simulink model "dedisp_sync"  (R2013b)
settings: Solver=FixedStepDiscrete  SolverMode=SingleTasking  StartTime=0.0  StopTime=10.0  RelTol=1e-3
undefined symbols (not defined in the file): pfb_coeff_gen_calc
libraries: xbsIndex_r4 x14646, casper_library_misc x70, casper_library_delays x55, dspsigops x16, xps_library x2, casper_library_pfbs x2
(part 53 of 146)

== system dedisp_sync/Parallel_Dedispersor_v5/Dedispersor_v2_4/detector_block_v212 ==
  Data : Inport
  Valid : Inport  Port=2
  Const1 : xbsIndex_r4/Constant  const=12  gui_display_data_type=Fixed-point  arith_type=Signed (2's comp)  n_bits=16  bin_pt=0  preci_type=Single  exp_width=8  frac_width=24  explicit_period=off  period=1  equ=P=C  opselect=C  inp2=PCIN>>17  opr=+  inp1=P  carry=CIN  dbl_ovrd=off  block_type=constant
  Counter1 : xbsIndex_r4/Counter  cnt_type=Free Running  cnt_to=Inf  operation=Up  start_count=0  cnt_by_val=1  arith_type=Unsigned  n_bits=4  bin_pt=0  load_pin=off  rst=off  en=on  explicit_period=on  period=1  dbl_ovrd=off  use_behavioral_HDL=off  implementation=Fabric  block_type=counter
  Delay1 : xbsIndex_r4/Delay  rst=off  infoeditControl=Selection of Reset will increase slice count due to use of real FFs and instead of SRLs  en=on  latency=13  dbl_ovrd=off  reg_retiming=on  block_type=delay
  Expression1 : xbsIndex_r4/Expression  expression=a & b  align_bp=on  en=off  latency=0  precision=Full  arith_type=Unsigned  n_bits=16  bin_pt=0  dbl_ovrd=off  block_type=expr
  Relational1 : xbsIndex_r4/Relational  mode=a=b  en=off  latency=0  dbl_ovrd=off  block_type=relational
  Out1 : Outport
  wires:
  Valid/1 -> Counter1/1, Expression1/2
  Counter1/1 -> Relational1/1
  Const1/1 -> Relational1/2
  Relational1/1 -> Expression1/1
  Data/1 -> Delay1/1
  Expression1/1 -> Delay1/2
  Delay1/1 -> Out1/1

== system dedisp_sync/Parallel_Dedispersor_v5/Dedispersor_v2_4/detector_block_v213 ==
  Data : Inport
  Valid : Inport  Port=2
  Const1 : xbsIndex_r4/Constant  const=13  gui_display_data_type=Fixed-point  arith_type=Signed (2's comp)  n_bits=16  bin_pt=0  preci_type=Single  exp_width=8  frac_width=24  explicit_period=off  period=1  equ=P=C  opselect=C  inp2=PCIN>>17  opr=+  inp1=P  carry=CIN  dbl_ovrd=off  block_type=constant
  Counter1 : xbsIndex_r4/Counter  cnt_type=Free Running  cnt_to=Inf  operation=Up  start_count=0  cnt_by_val=1  arith_type=Unsigned  n_bits=4  bin_pt=0  load_pin=off  rst=off  en=on  explicit_period=on  period=1  dbl_ovrd=off  use_behavioral_HDL=off  implementation=Fabric  block_type=counter
  Delay1 : xbsIndex_r4/Delay  rst=off  infoeditControl=Selection of Reset will increase slice count due to use of real FFs and instead of SRLs  en=on  latency=14  dbl_ovrd=off  reg_retiming=on  block_type=delay
  Expression1 : xbsIndex_r4/Expression  expression=a & b  align_bp=on  en=off  latency=0  precision=Full  arith_type=Unsigned  n_bits=16  bin_pt=0  dbl_ovrd=off  block_type=expr
  Relational1 : xbsIndex_r4/Relational  mode=a=b  en=off  latency=0  dbl_ovrd=off  block_type=relational
  Out1 : Outport
  wires:
  Valid/1 -> Counter1/1, Expression1/2
  Counter1/1 -> Relational1/1
  Const1/1 -> Relational1/2
  Relational1/1 -> Expression1/1
  Data/1 -> Delay1/1
  Expression1/1 -> Delay1/2
  Delay1/1 -> Out1/1

== system dedisp_sync/Parallel_Dedispersor_v5/Dedispersor_v2_4/detector_block_v214 ==
  Data : Inport
  Valid : Inport  Port=2
  Const1 : xbsIndex_r4/Constant  const=14  gui_display_data_type=Fixed-point  arith_type=Signed (2's comp)  n_bits=16  bin_pt=0  preci_type=Single  exp_width=8  frac_width=24  explicit_period=off  period=1  equ=P=C  opselect=C  inp2=PCIN>>17  opr=+  inp1=P  carry=CIN  dbl_ovrd=off  block_type=constant
  Counter1 : xbsIndex_r4/Counter  cnt_type=Free Running  cnt_to=Inf  operation=Up  start_count=0  cnt_by_val=1  arith_type=Unsigned  n_bits=4  bin_pt=0  load_pin=off  rst=off  en=on  explicit_period=on  period=1  dbl_ovrd=off  use_behavioral_HDL=off  implementation=Fabric  block_type=counter
  Delay1 : xbsIndex_r4/Delay  rst=off  infoeditControl=Selection of Reset will increase slice count due to use of real FFs and instead of SRLs  en=on  latency=15  dbl_ovrd=off  reg_retiming=on  block_type=delay
  Expression1 : xbsIndex_r4/Expression  expression=a & b  align_bp=on  en=off  latency=0  precision=Full  arith_type=Unsigned  n_bits=16  bin_pt=0  dbl_ovrd=off  block_type=expr
  Relational1 : xbsIndex_r4/Relational  mode=a=b  en=off  latency=0  dbl_ovrd=off  block_type=relational
  Out1 : Outport
  wires:
  Valid/1 -> Counter1/1, Expression1/2
  Counter1/1 -> Relational1/1
  Const1/1 -> Relational1/2
  Relational1/1 -> Expression1/1
  Data/1 -> Delay1/1
  Expression1/1 -> Delay1/2
  Delay1/1 -> Out1/1

== system dedisp_sync/Parallel_Dedispersor_v5/Dedispersor_v2_4/detector_block_v215 ==
  Data : Inport
  Valid : Inport  Port=2
  Const1 : xbsIndex_r4/Constant  const=15  gui_display_data_type=Fixed-point  arith_type=Signed (2's comp)  n_bits=16  bin_pt=0  preci_type=Single  exp_width=8  frac_width=24  explicit_period=off  period=1  equ=P=C  opselect=C  inp2=PCIN>>17  opr=+  inp1=P  carry=CIN  dbl_ovrd=off  block_type=constant
  Counter1 : xbsIndex_r4/Counter  cnt_type=Free Running  cnt_to=Inf  operation=Up  start_count=0  cnt_by_val=1  arith_type=Unsigned  n_bits=4  bin_pt=0  load_pin=off  rst=off  en=on  explicit_period=on  period=1  dbl_ovrd=off  use_behavioral_HDL=off  implementation=Fabric  block_type=counter
  Delay1 : xbsIndex_r4/Delay  rst=off  infoeditControl=Selection of Reset will increase slice count due to use of real FFs and instead of SRLs  en=on  latency=16  dbl_ovrd=off  reg_retiming=on  block_type=delay
  Expression1 : xbsIndex_r4/Expression  expression=a & b  align_bp=on  en=off  latency=0  precision=Full  arith_type=Unsigned  n_bits=16  bin_pt=0  dbl_ovrd=off  block_type=expr
  Relational1 : xbsIndex_r4/Relational  mode=a=b  en=off  latency=0  dbl_ovrd=off  block_type=relational
  Out1 : Outport
  wires:
  Valid/1 -> Counter1/1, Expression1/2
  Counter1/1 -> Relational1/1
  Const1/1 -> Relational1/2
  Relational1/1 -> Expression1/1
  Data/1 -> Delay1/1
  Expression1/1 -> Delay1/2
  Delay1/1 -> Out1/1

== system dedisp_sync/Parallel_Dedispersor_v5/Dedispersor_v2_4/detector_block_v22 ==
  Data : Inport
  Valid : Inport  Port=2
  Const1 : xbsIndex_r4/Constant  const=2  gui_display_data_type=Fixed-point  arith_type=Signed (2's comp)  n_bits=16  bin_pt=0  preci_type=Single  exp_width=8  frac_width=24  explicit_period=off  period=1  equ=P=C  opselect=C  inp2=PCIN>>17  opr=+  inp1=P  carry=CIN  dbl_ovrd=off  block_type=constant
  Counter1 : xbsIndex_r4/Counter  cnt_type=Free Running  cnt_to=Inf  operation=Up  start_count=0  cnt_by_val=1  arith_type=Unsigned  n_bits=4  bin_pt=0  load_pin=off  rst=off  en=on  explicit_period=on  period=1  dbl_ovrd=off  use_behavioral_HDL=off  implementation=Fabric  block_type=counter
  Delay1 : xbsIndex_r4/Delay  rst=off  infoeditControl=Selection of Reset will increase slice count due to use of real FFs and instead of SRLs  en=on  latency=3  dbl_ovrd=off  reg_retiming=on  block_type=delay
  Expression1 : xbsIndex_r4/Expression  expression=a & b  align_bp=on  en=off  latency=0  precision=Full  arith_type=Unsigned  n_bits=16  bin_pt=0  dbl_ovrd=off  block_type=expr
  Relational1 : xbsIndex_r4/Relational  mode=a=b  en=off  latency=0  dbl_ovrd=off  block_type=relational
  Out1 : Outport
  wires:
  Valid/1 -> Counter1/1, Expression1/2
  Counter1/1 -> Relational1/1
  Const1/1 -> Relational1/2
  Relational1/1 -> Expression1/1
  Data/1 -> Delay1/1
  Expression1/1 -> Delay1/2
  Delay1/1 -> Out1/1

== system dedisp_sync/Parallel_Dedispersor_v5/Dedispersor_v2_4/detector_block_v23 ==
  Data : Inport
  Valid : Inport  Port=2
  Const1 : xbsIndex_r4/Constant  const=3  gui_display_data_type=Fixed-point  arith_type=Signed (2's comp)  n_bits=16  bin_pt=0  preci_type=Single  exp_width=8  frac_width=24  explicit_period=off  period=1  equ=P=C  opselect=C  inp2=PCIN>>17  opr=+  inp1=P  carry=CIN  dbl_ovrd=off  block_type=constant
  Counter1 : xbsIndex_r4/Counter  cnt_type=Free Running  cnt_to=Inf  operation=Up  start_count=0  cnt_by_val=1  arith_type=Unsigned  n_bits=4  bin_pt=0  load_pin=off  rst=off  en=on  explicit_period=on  period=1  dbl_ovrd=off  use_behavioral_HDL=off  implementation=Fabric  block_type=counter
  Delay1 : xbsIndex_r4/Delay  rst=off  infoeditControl=Selection of Reset will increase slice count due to use of real FFs and instead of SRLs  en=on  latency=4  dbl_ovrd=off  reg_retiming=on  block_type=delay
  Expression1 : xbsIndex_r4/Expression  expression=a & b  align_bp=on  en=off  latency=0  precision=Full  arith_type=Unsigned  n_bits=16  bin_pt=0  dbl_ovrd=off  block_type=expr
  Relational1 : xbsIndex_r4/Relational  mode=a=b  en=off  latency=0  dbl_ovrd=off  block_type=relational
  Out1 : Outport
  wires:
  Valid/1 -> Counter1/1, Expression1/2
  Counter1/1 -> Relational1/1
  Const1/1 -> Relational1/2
  Relational1/1 -> Expression1/1
  Data/1 -> Delay1/1
  Expression1/1 -> Delay1/2
  Delay1/1 -> Out1/1

== system dedisp_sync/Parallel_Dedispersor_v5/Dedispersor_v2_4/detector_block_v24 ==
  Data : Inport
  Valid : Inport  Port=2
  Const1 : xbsIndex_r4/Constant  const=4  gui_display_data_type=Fixed-point  arith_type=Signed (2's comp)  n_bits=16  bin_pt=0  preci_type=Single  exp_width=8  frac_width=24  explicit_period=off  period=1  equ=P=C  opselect=C  inp2=PCIN>>17  opr=+  inp1=P  carry=CIN  dbl_ovrd=off  block_type=constant
  Counter1 : xbsIndex_r4/Counter  cnt_type=Free Running  cnt_to=Inf  operation=Up  start_count=0  cnt_by_val=1  arith_type=Unsigned  n_bits=4  bin_pt=0  load_pin=off  rst=off  en=on  explicit_period=on  period=1  dbl_ovrd=off  use_behavioral_HDL=off  implementation=Fabric  block_type=counter
  Delay1 : xbsIndex_r4/Delay  rst=off  infoeditControl=Selection of Reset will increase slice count due to use of real FFs and instead of SRLs  en=on  latency=5  dbl_ovrd=off  reg_retiming=on  block_type=delay
  Expression1 : xbsIndex_r4/Expression  expression=a & b  align_bp=on  en=off  latency=0  precision=Full  arith_type=Unsigned  n_bits=16  bin_pt=0  dbl_ovrd=off  block_type=expr
  Relational1 : xbsIndex_r4/Relational  mode=a=b  en=off  latency=0  dbl_ovrd=off  block_type=relational
  Out1 : Outport
  wires:
  Valid/1 -> Counter1/1, Expression1/2
  Counter1/1 -> Relational1/1
  Const1/1 -> Relational1/2
  Relational1/1 -> Expression1/1
  Data/1 -> Delay1/1
  Expression1/1 -> Delay1/2
  Delay1/1 -> Out1/1

== system dedisp_sync/Parallel_Dedispersor_v5/Dedispersor_v2_4/detector_block_v25 ==
  Data : Inport
  Valid : Inport  Port=2
  Const1 : xbsIndex_r4/Constant  const=5  gui_display_data_type=Fixed-point  arith_type=Signed (2's comp)  n_bits=16  bin_pt=0  preci_type=Single  exp_width=8  frac_width=24  explicit_period=off  period=1  equ=P=C  opselect=C  inp2=PCIN>>17  opr=+  inp1=P  carry=CIN  dbl_ovrd=off  block_type=constant
  Counter1 : xbsIndex_r4/Counter  cnt_type=Free Running  cnt_to=Inf  operation=Up  start_count=0  cnt_by_val=1  arith_type=Unsigned  n_bits=4  bin_pt=0  load_pin=off  rst=off  en=on  explicit_period=on  period=1  dbl_ovrd=off  use_behavioral_HDL=off  implementation=Fabric  block_type=counter
  Delay1 : xbsIndex_r4/Delay  rst=off  infoeditControl=Selection of Reset will increase slice count due to use of real FFs and instead of SRLs  en=on  latency=6  dbl_ovrd=off  reg_retiming=on  block_type=delay
  Expression1 : xbsIndex_r4/Expression  expression=a & b  align_bp=on  en=off  latency=0  precision=Full  arith_type=Unsigned  n_bits=16  bin_pt=0  dbl_ovrd=off  block_type=expr
  Relational1 : xbsIndex_r4/Relational  mode=a=b  en=off  latency=0  dbl_ovrd=off  block_type=relational
  Out1 : Outport
  wires:
  Valid/1 -> Counter1/1, Expression1/2
  Counter1/1 -> Relational1/1
  Const1/1 -> Relational1/2
  Relational1/1 -> Expression1/1
  Data/1 -> Delay1/1
  Expression1/1 -> Delay1/2
  Delay1/1 -> Out1/1

== system dedisp_sync/Parallel_Dedispersor_v5/Dedispersor_v2_4/detector_block_v26 ==
  Data : Inport
  Valid : Inport  Port=2
  Const1 : xbsIndex_r4/Constant  const=6  gui_display_data_type=Fixed-point  arith_type=Signed (2's comp)  n_bits=16  bin_pt=0  preci_type=Single  exp_width=8  frac_width=24  explicit_period=off  period=1  equ=P=C  opselect=C  inp2=PCIN>>17  opr=+  inp1=P  carry=CIN  dbl_ovrd=off  block_type=constant
  Counter1 : xbsIndex_r4/Counter  cnt_type=Free Running  cnt_to=Inf  operation=Up  start_count=0  cnt_by_val=1  arith_type=Unsigned  n_bits=4  bin_pt=0  load_pin=off  rst=off  en=on  explicit_period=on  period=1  dbl_ovrd=off  use_behavioral_HDL=off  implementation=Fabric  block_type=counter
  Delay1 : xbsIndex_r4/Delay  rst=off  infoeditControl=Selection of Reset will increase slice count due to use of real FFs and instead of SRLs  en=on  latency=7  dbl_ovrd=off  reg_retiming=on  block_type=delay
  Expression1 : xbsIndex_r4/Expression  expression=a & b  align_bp=on  en=off  latency=0  precision=Full  arith_type=Unsigned  n_bits=16  bin_pt=0  dbl_ovrd=off  block_type=expr
  Relational1 : xbsIndex_r4/Relational  mode=a=b  en=off  latency=0  dbl_ovrd=off  block_type=relational
  Out1 : Outport
  wires:
  Valid/1 -> Counter1/1, Expression1/2
  Counter1/1 -> Relational1/1
  Const1/1 -> Relational1/2
  Relational1/1 -> Expression1/1
  Data/1 -> Delay1/1
  Expression1/1 -> Delay1/2
  Delay1/1 -> Out1/1

== system dedisp_sync/Parallel_Dedispersor_v5/Dedispersor_v2_4/detector_block_v27 ==
  Data : Inport
  Valid : Inport  Port=2
  Const1 : xbsIndex_r4/Constant  const=7  gui_display_data_type=Fixed-point  arith_type=Signed (2's comp)  n_bits=16  bin_pt=0  preci_type=Single  exp_width=8  frac_width=24  explicit_period=off  period=1  equ=P=C  opselect=C  inp2=PCIN>>17  opr=+  inp1=P  carry=CIN  dbl_ovrd=off  block_type=constant
  Counter1 : xbsIndex_r4/Counter  cnt_type=Free Running  cnt_to=Inf  operation=Up  start_count=0  cnt_by_val=1  arith_type=Unsigned  n_bits=4  bin_pt=0  load_pin=off  rst=off  en=on  explicit_period=on  period=1  dbl_ovrd=off  use_behavioral_HDL=off  implementation=Fabric  block_type=counter
  Delay1 : xbsIndex_r4/Delay  rst=off  infoeditControl=Selection of Reset will increase slice count due to use of real FFs and instead of SRLs  en=on  latency=8  dbl_ovrd=off  reg_retiming=on  block_type=delay
  Expression1 : xbsIndex_r4/Expression  expression=a & b  align_bp=on  en=off  latency=0  precision=Full  arith_type=Unsigned  n_bits=16  bin_pt=0  dbl_ovrd=off  block_type=expr
  Relational1 : xbsIndex_r4/Relational  mode=a=b  en=off  latency=0  dbl_ovrd=off  block_type=relational
  Out1 : Outport
  wires:
  Valid/1 -> Counter1/1, Expression1/2
  Counter1/1 -> Relational1/1
  Const1/1 -> Relational1/2
  Relational1/1 -> Expression1/1
  Data/1 -> Delay1/1
  Expression1/1 -> Delay1/2
  Delay1/1 -> Out1/1

== system dedisp_sync/Parallel_Dedispersor_v5/Dedispersor_v2_4/detector_block_v28 ==
  Data : Inport
  Valid : Inport  Port=2
  Const1 : xbsIndex_r4/Constant  const=8  gui_display_data_type=Fixed-point  arith_type=Signed (2's comp)  n_bits=16  bin_pt=0  preci_type=Single  exp_width=8  frac_width=24  explicit_period=off  period=1  equ=P=C  opselect=C  inp2=PCIN>>17  opr=+  inp1=P  carry=CIN  dbl_ovrd=off  block_type=constant
  Counter1 : xbsIndex_r4/Counter  cnt_type=Free Running  cnt_to=Inf  operation=Up  start_count=0  cnt_by_val=1  arith_type=Unsigned  n_bits=4  bin_pt=0  load_pin=off  rst=off  en=on  explicit_period=on  period=1  dbl_ovrd=off  use_behavioral_HDL=off  implementation=Fabric  block_type=counter
  Delay1 : xbsIndex_r4/Delay  rst=off  infoeditControl=Selection of Reset will increase slice count due to use of real FFs and instead of SRLs  en=on  latency=9  dbl_ovrd=off  reg_retiming=on  block_type=delay
  Expression1 : xbsIndex_r4/Expression  expression=a & b  align_bp=on  en=off  latency=0  precision=Full  arith_type=Unsigned  n_bits=16  bin_pt=0  dbl_ovrd=off  block_type=expr
  Relational1 : xbsIndex_r4/Relational  mode=a=b  en=off  latency=0  dbl_ovrd=off  block_type=relational
  Out1 : Outport
  wires:
  Valid/1 -> Counter1/1, Expression1/2
  Counter1/1 -> Relational1/1
  Const1/1 -> Relational1/2
  Relational1/1 -> Expression1/1
  Data/1 -> Delay1/1
  Expression1/1 -> Delay1/2
  Delay1/1 -> Out1/1

== system dedisp_sync/Parallel_Dedispersor_v5/Dedispersor_v2_4/detector_block_v29 ==
  Data : Inport
  Valid : Inport  Port=2
  Const1 : xbsIndex_r4/Constant  const=9  gui_display_data_type=Fixed-point  arith_type=Signed (2's comp)  n_bits=16  bin_pt=0  preci_type=Single  exp_width=8  frac_width=24  explicit_period=off  period=1  equ=P=C  opselect=C  inp2=PCIN>>17  opr=+  inp1=P  carry=CIN  dbl_ovrd=off  block_type=constant
  Counter1 : xbsIndex_r4/Counter  cnt_type=Free Running  cnt_to=Inf  operation=Up  start_count=0  cnt_by_val=1  arith_type=Unsigned  n_bits=4  bin_pt=0  load_pin=off  rst=off  en=on  explicit_period=on  period=1  dbl_ovrd=off  use_behavioral_HDL=off  implementation=Fabric  block_type=counter
  Delay1 : xbsIndex_r4/Delay  rst=off  infoeditControl=Selection of Reset will increase slice count due to use of real FFs and instead of SRLs  en=on  latency=10  dbl_ovrd=off  reg_retiming=on  block_type=delay
  Expression1 : xbsIndex_r4/Expression  expression=a & b  align_bp=on  en=off  latency=0  precision=Full  arith_type=Unsigned  n_bits=16  bin_pt=0  dbl_ovrd=off  block_type=expr
  Relational1 : xbsIndex_r4/Relational  mode=a=b  en=off  latency=0  dbl_ovrd=off  block_type=relational
  Out1 : Outport
  wires:
  Valid/1 -> Counter1/1, Expression1/2
  Counter1/1 -> Relational1/1
  Const1/1 -> Relational1/2
  Relational1/1 -> Expression1/1
  Data/1 -> Delay1/1
  Expression1/1 -> Delay1/2
  Delay1/1 -> Out1/1

== system dedisp_sync/Parallel_Dedispersor_v6/Dedispersor_v2_1/detector_block_v2 ==
  Data : Inport
  Valid : Inport  Port=2
  Const1 : xbsIndex_r4/Constant  const=0  gui_display_data_type=Fixed-point  arith_type=Signed (2's comp)  n_bits=16  bin_pt=0  preci_type=Single  exp_width=8  frac_width=24  explicit_period=off  period=1  equ=P=C  opselect=C  inp2=PCIN>>17  opr=+  inp1=P  carry=CIN  dbl_ovrd=off  block_type=constant
  Counter1 : xbsIndex_r4/Counter  cnt_type=Free Running  cnt_to=Inf  operation=Up  start_count=0  cnt_by_val=1  arith_type=Unsigned  n_bits=4  bin_pt=0  load_pin=off  rst=off  en=on  explicit_period=on  period=1  dbl_ovrd=off  use_behavioral_HDL=off  implementation=Fabric  block_type=counter
  Delay1 : xbsIndex_r4/Delay  rst=off  infoeditControl=Selection of Reset will increase slice count due to use of real FFs and instead of SRLs  en=on  latency=1  dbl_ovrd=off  reg_retiming=on  block_type=delay
  Expression1 : xbsIndex_r4/Expression  expression=a & b  align_bp=on  en=off  latency=0  precision=Full  arith_type=Unsigned  n_bits=16  bin_pt=0  dbl_ovrd=off  block_type=expr
  Relational1 : xbsIndex_r4/Relational  mode=a=b  en=off  latency=0  dbl_ovrd=off  block_type=relational
  Out1 : Outport
  wires:
  Valid/1 -> Counter1/1, Expression1/2
  Counter1/1 -> Relational1/1
  Const1/1 -> Relational1/2
  Relational1/1 -> Expression1/1
  Data/1 -> Delay1/1
  Expression1/1 -> Delay1/2
  Delay1/1 -> Out1/1

== system dedisp_sync/Parallel_Dedispersor_v6/Dedispersor_v2_1/detector_block_v21 ==
  Data : Inport
  Valid : Inport  Port=2
  Const1 : xbsIndex_r4/Constant  const=1  gui_display_data_type=Fixed-point  arith_type=Signed (2's comp)  n_bits=16  bin_pt=0  preci_type=Single  exp_width=8  frac_width=24  explicit_period=off  period=1  equ=P=C  opselect=C  inp2=PCIN>>17  opr=+  inp1=P  carry=CIN  dbl_ovrd=off  block_type=constant
  Counter1 : xbsIndex_r4/Counter  cnt_type=Free Running  cnt_to=Inf  operation=Up  start_count=0  cnt_by_val=1  arith_type=Unsigned  n_bits=4  bin_pt=0  load_pin=off  rst=off  en=on  explicit_period=on  period=1  dbl_ovrd=off  use_behavioral_HDL=off  implementation=Fabric  block_type=counter
  Delay1 : xbsIndex_r4/Delay  rst=off  infoeditControl=Selection of Reset will increase slice count due to use of real FFs and instead of SRLs  en=on  latency=2  dbl_ovrd=off  reg_retiming=on  block_type=delay
  Expression1 : xbsIndex_r4/Expression  expression=a & b  align_bp=on  en=off  latency=0  precision=Full  arith_type=Unsigned  n_bits=16  bin_pt=0  dbl_ovrd=off  block_type=expr
  Relational1 : xbsIndex_r4/Relational  mode=a=b  en=off  latency=0  dbl_ovrd=off  block_type=relational
  Out1 : Outport
  wires:
  Valid/1 -> Counter1/1, Expression1/2
  Counter1/1 -> Relational1/1
  Const1/1 -> Relational1/2
  Relational1/1 -> Expression1/1
  Data/1 -> Delay1/1
  Expression1/1 -> Delay1/2
  Delay1/1 -> Out1/1

== system dedisp_sync/Parallel_Dedispersor_v6/Dedispersor_v2_1/detector_block_v210 ==
  Data : Inport
  Valid : Inport  Port=2
  Const1 : xbsIndex_r4/Constant  const=10  gui_display_data_type=Fixed-point  arith_type=Signed (2's comp)  n_bits=16  bin_pt=0  preci_type=Single  exp_width=8  frac_width=24  explicit_period=off  period=1  equ=P=C  opselect=C  inp2=PCIN>>17  opr=+  inp1=P  carry=CIN  dbl_ovrd=off  block_type=constant
  Counter1 : xbsIndex_r4/Counter  cnt_type=Free Running  cnt_to=Inf  operation=Up  start_count=0  cnt_by_val=1  arith_type=Unsigned  n_bits=4  bin_pt=0  load_pin=off  rst=off  en=on  explicit_period=on  period=1  dbl_ovrd=off  use_behavioral_HDL=off  implementation=Fabric  block_type=counter
  Delay1 : xbsIndex_r4/Delay  rst=off  infoeditControl=Selection of Reset will increase slice count due to use of real FFs and instead of SRLs  en=on  latency=11  dbl_ovrd=off  reg_retiming=on  block_type=delay
  Expression1 : xbsIndex_r4/Expression  expression=a & b  align_bp=on  en=off  latency=0  precision=Full  arith_type=Unsigned  n_bits=16  bin_pt=0  dbl_ovrd=off  block_type=expr
  Relational1 : xbsIndex_r4/Relational  mode=a=b  en=off  latency=0  dbl_ovrd=off  block_type=relational
  Out1 : Outport
  wires:
  Valid/1 -> Counter1/1, Expression1/2
  Counter1/1 -> Relational1/1
  Const1/1 -> Relational1/2
  Relational1/1 -> Expression1/1
  Data/1 -> Delay1/1
  Expression1/1 -> Delay1/2
  Delay1/1 -> Out1/1

== system dedisp_sync/Parallel_Dedispersor_v6/Dedispersor_v2_1/detector_block_v211 ==
  Data : Inport
  Valid : Inport  Port=2
  Const1 : xbsIndex_r4/Constant  const=11  gui_display_data_type=Fixed-point  arith_type=Signed (2's comp)  n_bits=16  bin_pt=0  preci_type=Single  exp_width=8  frac_width=24  explicit_period=off  period=1  equ=P=C  opselect=C  inp2=PCIN>>17  opr=+  inp1=P  carry=CIN  dbl_ovrd=off  block_type=constant
  Counter1 : xbsIndex_r4/Counter  cnt_type=Free Running  cnt_to=Inf  operation=Up  start_count=0  cnt_by_val=1  arith_type=Unsigned  n_bits=4  bin_pt=0  load_pin=off  rst=off  en=on  explicit_period=on  period=1  dbl_ovrd=off  use_behavioral_HDL=off  implementation=Fabric  block_type=counter
  Delay1 : xbsIndex_r4/Delay  rst=off  infoeditControl=Selection of Reset will increase slice count due to use of real FFs and instead of SRLs  en=on  latency=12  dbl_ovrd=off  reg_retiming=on  block_type=delay
  Expression1 : xbsIndex_r4/Expression  expression=a & b  align_bp=on  en=off  latency=0  precision=Full  arith_type=Unsigned  n_bits=16  bin_pt=0  dbl_ovrd=off  block_type=expr
  Relational1 : xbsIndex_r4/Relational  mode=a=b  en=off  latency=0  dbl_ovrd=off  block_type=relational
  Out1 : Outport
  wires:
  Valid/1 -> Counter1/1, Expression1/2
  Counter1/1 -> Relational1/1
  Const1/1 -> Relational1/2
  Relational1/1 -> Expression1/1
  Data/1 -> Delay1/1
  Expression1/1 -> Delay1/2
  Delay1/1 -> Out1/1

== system dedisp_sync/Parallel_Dedispersor_v6/Dedispersor_v2_1/detector_block_v212 ==
  Data : Inport
  Valid : Inport  Port=2
  Const1 : xbsIndex_r4/Constant  const=12  gui_display_data_type=Fixed-point  arith_type=Signed (2's comp)  n_bits=16  bin_pt=0  preci_type=Single  exp_width=8  frac_width=24  explicit_period=off  period=1  equ=P=C  opselect=C  inp2=PCIN>>17  opr=+  inp1=P  carry=CIN  dbl_ovrd=off  block_type=constant
  Counter1 : xbsIndex_r4/Counter  cnt_type=Free Running  cnt_to=Inf  operation=Up  start_count=0  cnt_by_val=1  arith_type=Unsigned  n_bits=4  bin_pt=0  load_pin=off  rst=off  en=on  explicit_period=on  period=1  dbl_ovrd=off  use_behavioral_HDL=off  implementation=Fabric  block_type=counter
  Delay1 : xbsIndex_r4/Delay  rst=off  infoeditControl=Selection of Reset will increase slice count due to use of real FFs and instead of SRLs  en=on  latency=13  dbl_ovrd=off  reg_retiming=on  block_type=delay
  Expression1 : xbsIndex_r4/Expression  expression=a & b  align_bp=on  en=off  latency=0  precision=Full  arith_type=Unsigned  n_bits=16  bin_pt=0  dbl_ovrd=off  block_type=expr
  Relational1 : xbsIndex_r4/Relational  mode=a=b  en=off  latency=0  dbl_ovrd=off  block_type=relational
  Out1 : Outport
  wires:
  Valid/1 -> Counter1/1, Expression1/2
  Counter1/1 -> Relational1/1
  Const1/1 -> Relational1/2
  Relational1/1 -> Expression1/1
  Data/1 -> Delay1/1
  Expression1/1 -> Delay1/2
  Delay1/1 -> Out1/1

== system dedisp_sync/Parallel_Dedispersor_v6/Dedispersor_v2_1/detector_block_v213 ==
  Data : Inport
  Valid : Inport  Port=2
  Const1 : xbsIndex_r4/Constant  const=13  gui_display_data_type=Fixed-point  arith_type=Signed (2's comp)  n_bits=16  bin_pt=0  preci_type=Single  exp_width=8  frac_width=24  explicit_period=off  period=1  equ=P=C  opselect=C  inp2=PCIN>>17  opr=+  inp1=P  carry=CIN  dbl_ovrd=off  block_type=constant
  Counter1 : xbsIndex_r4/Counter  cnt_type=Free Running  cnt_to=Inf  operation=Up  start_count=0  cnt_by_val=1  arith_type=Unsigned  n_bits=4  bin_pt=0  load_pin=off  rst=off  en=on  explicit_period=on  period=1  dbl_ovrd=off  use_behavioral_HDL=off  implementation=Fabric  block_type=counter
  Delay1 : xbsIndex_r4/Delay  rst=off  infoeditControl=Selection of Reset will increase slice count due to use of real FFs and instead of SRLs  en=on  latency=14  dbl_ovrd=off  reg_retiming=on  block_type=delay
  Expression1 : xbsIndex_r4/Expression  expression=a & b  align_bp=on  en=off  latency=0  precision=Full  arith_type=Unsigned  n_bits=16  bin_pt=0  dbl_ovrd=off  block_type=expr
  Relational1 : xbsIndex_r4/Relational  mode=a=b  en=off  latency=0  dbl_ovrd=off  block_type=relational
  Out1 : Outport
  wires:
  Valid/1 -> Counter1/1, Expression1/2
  Counter1/1 -> Relational1/1
  Const1/1 -> Relational1/2
  Relational1/1 -> Expression1/1
  Data/1 -> Delay1/1
  Expression1/1 -> Delay1/2
  Delay1/1 -> Out1/1

== system dedisp_sync/Parallel_Dedispersor_v6/Dedispersor_v2_1/detector_block_v214 ==
  Data : Inport
  Valid : Inport  Port=2
  Const1 : xbsIndex_r4/Constant  const=14  gui_display_data_type=Fixed-point  arith_type=Signed (2's comp)  n_bits=16  bin_pt=0  preci_type=Single  exp_width=8  frac_width=24  explicit_period=off  period=1  equ=P=C  opselect=C  inp2=PCIN>>17  opr=+  inp1=P  carry=CIN  dbl_ovrd=off  block_type=constant
  Counter1 : xbsIndex_r4/Counter  cnt_type=Free Running  cnt_to=Inf  operation=Up  start_count=0  cnt_by_val=1  arith_type=Unsigned  n_bits=4  bin_pt=0  load_pin=off  rst=off  en=on  explicit_period=on  period=1  dbl_ovrd=off  use_behavioral_HDL=off  implementation=Fabric  block_type=counter
  Delay1 : xbsIndex_r4/Delay  rst=off  infoeditControl=Selection of Reset will increase slice count due to use of real FFs and instead of SRLs  en=on  latency=15  dbl_ovrd=off  reg_retiming=on  block_type=delay
  Expression1 : xbsIndex_r4/Expression  expression=a & b  align_bp=on  en=off  latency=0  precision=Full  arith_type=Unsigned  n_bits=16  bin_pt=0  dbl_ovrd=off  block_type=expr
  Relational1 : xbsIndex_r4/Relational  mode=a=b  en=off  latency=0  dbl_ovrd=off  block_type=relational
  Out1 : Outport
  wires:
  Valid/1 -> Counter1/1, Expression1/2
  Counter1/1 -> Relational1/1
  Const1/1 -> Relational1/2
  Relational1/1 -> Expression1/1
  Data/1 -> Delay1/1
  Expression1/1 -> Delay1/2
  Delay1/1 -> Out1/1

== system dedisp_sync/Parallel_Dedispersor_v6/Dedispersor_v2_1/detector_block_v215 ==
  Data : Inport
  Valid : Inport  Port=2
  Const1 : xbsIndex_r4/Constant  const=15  gui_display_data_type=Fixed-point  arith_type=Signed (2's comp)  n_bits=16  bin_pt=0  preci_type=Single  exp_width=8  frac_width=24  explicit_period=off  period=1  equ=P=C  opselect=C  inp2=PCIN>>17  opr=+  inp1=P  carry=CIN  dbl_ovrd=off  block_type=constant
  Counter1 : xbsIndex_r4/Counter  cnt_type=Free Running  cnt_to=Inf  operation=Up  start_count=0  cnt_by_val=1  arith_type=Unsigned  n_bits=4  bin_pt=0  load_pin=off  rst=off  en=on  explicit_period=on  period=1  dbl_ovrd=off  use_behavioral_HDL=off  implementation=Fabric  block_type=counter
  Delay1 : xbsIndex_r4/Delay  rst=off  infoeditControl=Selection of Reset will increase slice count due to use of real FFs and instead of SRLs  en=on  latency=16  dbl_ovrd=off  reg_retiming=on  block_type=delay
  Expression1 : xbsIndex_r4/Expression  expression=a & b  align_bp=on  en=off  latency=0  precision=Full  arith_type=Unsigned  n_bits=16  bin_pt=0  dbl_ovrd=off  block_type=expr
  Relational1 : xbsIndex_r4/Relational  mode=a=b  en=off  latency=0  dbl_ovrd=off  block_type=relational
  Out1 : Outport
  wires:
  Valid/1 -> Counter1/1, Expression1/2
  Counter1/1 -> Relational1/1
  Const1/1 -> Relational1/2
  Relational1/1 -> Expression1/1
  Data/1 -> Delay1/1
  Expression1/1 -> Delay1/2
  Delay1/1 -> Out1/1

== system dedisp_sync/Parallel_Dedispersor_v6/Dedispersor_v2_1/detector_block_v22 ==
  Data : Inport
  Valid : Inport  Port=2
  Const1 : xbsIndex_r4/Constant  const=2  gui_display_data_type=Fixed-point  arith_type=Signed (2's comp)  n_bits=16  bin_pt=0  preci_type=Single  exp_width=8  frac_width=24  explicit_period=off  period=1  equ=P=C  opselect=C  inp2=PCIN>>17  opr=+  inp1=P  carry=CIN  dbl_ovrd=off  block_type=constant
  Counter1 : xbsIndex_r4/Counter  cnt_type=Free Running  cnt_to=Inf  operation=Up  start_count=0  cnt_by_val=1  arith_type=Unsigned  n_bits=4  bin_pt=0  load_pin=off  rst=off  en=on  explicit_period=on  period=1  dbl_ovrd=off  use_behavioral_HDL=off  implementation=Fabric  block_type=counter
  Delay1 : xbsIndex_r4/Delay  rst=off  infoeditControl=Selection of Reset will increase slice count due to use of real FFs and instead of SRLs  en=on  latency=3  dbl_ovrd=off  reg_retiming=on  block_type=delay
  Expression1 : xbsIndex_r4/Expression  expression=a & b  align_bp=on  en=off  latency=0  precision=Full  arith_type=Unsigned  n_bits=16  bin_pt=0  dbl_ovrd=off  block_type=expr
  Relational1 : xbsIndex_r4/Relational  mode=a=b  en=off  latency=0  dbl_ovrd=off  block_type=relational
  Out1 : Outport
  wires:
  Valid/1 -> Counter1/1, Expression1/2
  Counter1/1 -> Relational1/1
  Const1/1 -> Relational1/2
  Relational1/1 -> Expression1/1
  Data/1 -> Delay1/1
  Expression1/1 -> Delay1/2
  Delay1/1 -> Out1/1

== system dedisp_sync/Parallel_Dedispersor_v6/Dedispersor_v2_1/detector_block_v23 ==
  Data : Inport
  Valid : Inport  Port=2
  Const1 : xbsIndex_r4/Constant  const=3  gui_display_data_type=Fixed-point  arith_type=Signed (2's comp)  n_bits=16  bin_pt=0  preci_type=Single  exp_width=8  frac_width=24  explicit_period=off  period=1  equ=P=C  opselect=C  inp2=PCIN>>17  opr=+  inp1=P  carry=CIN  dbl_ovrd=off  block_type=constant
  Counter1 : xbsIndex_r4/Counter  cnt_type=Free Running  cnt_to=Inf  operation=Up  start_count=0  cnt_by_val=1  arith_type=Unsigned  n_bits=4  bin_pt=0  load_pin=off  rst=off  en=on  explicit_period=on  period=1  dbl_ovrd=off  use_behavioral_HDL=off  implementation=Fabric  block_type=counter
  Delay1 : xbsIndex_r4/Delay  rst=off  infoeditControl=Selection of Reset will increase slice count due to use of real FFs and instead of SRLs  en=on  latency=4  dbl_ovrd=off  reg_retiming=on  block_type=delay
  Expression1 : xbsIndex_r4/Expression  expression=a & b  align_bp=on  en=off  latency=0  precision=Full  arith_type=Unsigned  n_bits=16  bin_pt=0  dbl_ovrd=off  block_type=expr
  Relational1 : xbsIndex_r4/Relational  mode=a=b  en=off  latency=0  dbl_ovrd=off  block_type=relational
  Out1 : Outport
  wires:
  Valid/1 -> Counter1/1, Expression1/2
  Counter1/1 -> Relational1/1
  Const1/1 -> Relational1/2
  Relational1/1 -> Expression1/1
  Data/1 -> Delay1/1
  Expression1/1 -> Delay1/2
  Delay1/1 -> Out1/1

== system dedisp_sync/Parallel_Dedispersor_v6/Dedispersor_v2_1/detector_block_v24 ==
  Data : Inport
  Valid : Inport  Port=2
  Const1 : xbsIndex_r4/Constant  const=4  gui_display_data_type=Fixed-point  arith_type=Signed (2's comp)  n_bits=16  bin_pt=0  preci_type=Single  exp_width=8  frac_width=24  explicit_period=off  period=1  equ=P=C  opselect=C  inp2=PCIN>>17  opr=+  inp1=P  carry=CIN  dbl_ovrd=off  block_type=constant
  Counter1 : xbsIndex_r4/Counter  cnt_type=Free Running  cnt_to=Inf  operation=Up  start_count=0  cnt_by_val=1  arith_type=Unsigned  n_bits=4  bin_pt=0  load_pin=off  rst=off  en=on  explicit_period=on  period=1  dbl_ovrd=off  use_behavioral_HDL=off  implementation=Fabric  block_type=counter
  Delay1 : xbsIndex_r4/Delay  rst=off  infoeditControl=Selection of Reset will increase slice count due to use of real FFs and instead of SRLs  en=on  latency=5  dbl_ovrd=off  reg_retiming=on  block_type=delay
  Expression1 : xbsIndex_r4/Expression  expression=a & b  align_bp=on  en=off  latency=0  precision=Full  arith_type=Unsigned  n_bits=16  bin_pt=0  dbl_ovrd=off  block_type=expr
  Relational1 : xbsIndex_r4/Relational  mode=a=b  en=off  latency=0  dbl_ovrd=off  block_type=relational
  Out1 : Outport
  wires:
  Valid/1 -> Counter1/1, Expression1/2
  Counter1/1 -> Relational1/1
  Const1/1 -> Relational1/2
  Relational1/1 -> Expression1/1
  Data/1 -> Delay1/1
  Expression1/1 -> Delay1/2
  Delay1/1 -> Out1/1

== system dedisp_sync/Parallel_Dedispersor_v6/Dedispersor_v2_1/detector_block_v25 ==
  Data : Inport
  Valid : Inport  Port=2
  Const1 : xbsIndex_r4/Constant  const=5  gui_display_data_type=Fixed-point  arith_type=Signed (2's comp)  n_bits=16  bin_pt=0  preci_type=Single  exp_width=8  frac_width=24  explicit_period=off  period=1  equ=P=C  opselect=C  inp2=PCIN>>17  opr=+  inp1=P  carry=CIN  dbl_ovrd=off  block_type=constant
  Counter1 : xbsIndex_r4/Counter  cnt_type=Free Running  cnt_to=Inf  operation=Up  start_count=0  cnt_by_val=1  arith_type=Unsigned  n_bits=4  bin_pt=0  load_pin=off  rst=off  en=on  explicit_period=on  period=1  dbl_ovrd=off  use_behavioral_HDL=off  implementation=Fabric  block_type=counter
  Delay1 : xbsIndex_r4/Delay  rst=off  infoeditControl=Selection of Reset will increase slice count due to use of real FFs and instead of SRLs  en=on  latency=6  dbl_ovrd=off  reg_retiming=on  block_type=delay
  Expression1 : xbsIndex_r4/Expression  expression=a & b  align_bp=on  en=off  latency=0  precision=Full  arith_type=Unsigned  n_bits=16  bin_pt=0  dbl_ovrd=off  block_type=expr
  Relational1 : xbsIndex_r4/Relational  mode=a=b  en=off  latency=0  dbl_ovrd=off  block_type=relational
  Out1 : Outport
  wires:
  Valid/1 -> Counter1/1, Expression1/2
  Counter1/1 -> Relational1/1
  Const1/1 -> Relational1/2
  Relational1/1 -> Expression1/1
  Data/1 -> Delay1/1
  Expression1/1 -> Delay1/2
  Delay1/1 -> Out1/1

== system dedisp_sync/Parallel_Dedispersor_v6/Dedispersor_v2_1/detector_block_v26 ==
  Data : Inport
  Valid : Inport  Port=2
  Const1 : xbsIndex_r4/Constant  const=6  gui_display_data_type=Fixed-point  arith_type=Signed (2's comp)  n_bits=16  bin_pt=0  preci_type=Single  exp_width=8  frac_width=24  explicit_period=off  period=1  equ=P=C  opselect=C  inp2=PCIN>>17  opr=+  inp1=P  carry=CIN  dbl_ovrd=off  block_type=constant
  Counter1 : xbsIndex_r4/Counter  cnt_type=Free Running  cnt_to=Inf  operation=Up  start_count=0  cnt_by_val=1  arith_type=Unsigned  n_bits=4  bin_pt=0  load_pin=off  rst=off  en=on  explicit_period=on  period=1  dbl_ovrd=off  use_behavioral_HDL=off  implementation=Fabric  block_type=counter
  Delay1 : xbsIndex_r4/Delay  rst=off  infoeditControl=Selection of Reset will increase slice count due to use of real FFs and instead of SRLs  en=on  latency=7  dbl_ovrd=off  reg_retiming=on  block_type=delay
  Expression1 : xbsIndex_r4/Expression  expression=a & b  align_bp=on  en=off  latency=0  precision=Full  arith_type=Unsigned  n_bits=16  bin_pt=0  dbl_ovrd=off  block_type=expr
  Relational1 : xbsIndex_r4/Relational  mode=a=b  en=off  latency=0  dbl_ovrd=off  block_type=relational
  Out1 : Outport
  wires:
  Valid/1 -> Counter1/1, Expression1/2
  Counter1/1 -> Relational1/1
  Const1/1 -> Relational1/2
  Relational1/1 -> Expression1/1
  Data/1 -> Delay1/1
  Expression1/1 -> Delay1/2
  Delay1/1 -> Out1/1

== system dedisp_sync/Parallel_Dedispersor_v6/Dedispersor_v2_1/detector_block_v27 ==
  Data : Inport
  Valid : Inport  Port=2
  Const1 : xbsIndex_r4/Constant  const=7  gui_display_data_type=Fixed-point  arith_type=Signed (2's comp)  n_bits=16  bin_pt=0  preci_type=Single  exp_width=8  frac_width=24  explicit_period=off  period=1  equ=P=C  opselect=C  inp2=PCIN>>17  opr=+  inp1=P  carry=CIN  dbl_ovrd=off  block_type=constant
  Counter1 : xbsIndex_r4/Counter  cnt_type=Free Running  cnt_to=Inf  operation=Up  start_count=0  cnt_by_val=1  arith_type=Unsigned  n_bits=4  bin_pt=0  load_pin=off  rst=off  en=on  explicit_period=on  period=1  dbl_ovrd=off  use_behavioral_HDL=off  implementation=Fabric  block_type=counter
  Delay1 : xbsIndex_r4/Delay  rst=off  infoeditControl=Selection of Reset will increase slice count due to use of real FFs and instead of SRLs  en=on  latency=8  dbl_ovrd=off  reg_retiming=on  block_type=delay
  Expression1 : xbsIndex_r4/Expression  expression=a & b  align_bp=on  en=off  latency=0  precision=Full  arith_type=Unsigned  n_bits=16  bin_pt=0  dbl_ovrd=off  block_type=expr
  Relational1 : xbsIndex_r4/Relational  mode=a=b  en=off  latency=0  dbl_ovrd=off  block_type=relational
  Out1 : Outport
  wires:
  Valid/1 -> Counter1/1, Expression1/2
  Counter1/1 -> Relational1/1
  Const1/1 -> Relational1/2
  Relational1/1 -> Expression1/1
  Data/1 -> Delay1/1
  Expression1/1 -> Delay1/2
  Delay1/1 -> Out1/1

== system dedisp_sync/Parallel_Dedispersor_v6/Dedispersor_v2_1/detector_block_v28 ==
  Data : Inport
  Valid : Inport  Port=2
  Const1 : xbsIndex_r4/Constant  const=8  gui_display_data_type=Fixed-point  arith_type=Signed (2's comp)  n_bits=16  bin_pt=0  preci_type=Single  exp_width=8  frac_width=24  explicit_period=off  period=1  equ=P=C  opselect=C  inp2=PCIN>>17  opr=+  inp1=P  carry=CIN  dbl_ovrd=off  block_type=constant
  Counter1 : xbsIndex_r4/Counter  cnt_type=Free Running  cnt_to=Inf  operation=Up  start_count=0  cnt_by_val=1  arith_type=Unsigned  n_bits=4  bin_pt=0  load_pin=off  rst=off  en=on  explicit_period=on  period=1  dbl_ovrd=off  use_behavioral_HDL=off  implementation=Fabric  block_type=counter
  Delay1 : xbsIndex_r4/Delay  rst=off  infoeditControl=Selection of Reset will increase slice count due to use of real FFs and instead of SRLs  en=on  latency=9  dbl_ovrd=off  reg_retiming=on  block_type=delay
  Expression1 : xbsIndex_r4/Expression  expression=a & b  align_bp=on  en=off  latency=0  precision=Full  arith_type=Unsigned  n_bits=16  bin_pt=0  dbl_ovrd=off  block_type=expr
  Relational1 : xbsIndex_r4/Relational  mode=a=b  en=off  latency=0  dbl_ovrd=off  block_type=relational
  Out1 : Outport
  wires:
  Valid/1 -> Counter1/1, Expression1/2
  Counter1/1 -> Relational1/1
  Const1/1 -> Relational1/2
  Relational1/1 -> Expression1/1
  Data/1 -> Delay1/1
  Expression1/1 -> Delay1/2
  Delay1/1 -> Out1/1

== system dedisp_sync/Parallel_Dedispersor_v6/Dedispersor_v2_1/detector_block_v29 ==
  Data : Inport
  Valid : Inport  Port=2
  Const1 : xbsIndex_r4/Constant  const=9  gui_display_data_type=Fixed-point  arith_type=Signed (2's comp)  n_bits=16  bin_pt=0  preci_type=Single  exp_width=8  frac_width=24  explicit_period=off  period=1  equ=P=C  opselect=C  inp2=PCIN>>17  opr=+  inp1=P  carry=CIN  dbl_ovrd=off  block_type=constant
  Counter1 : xbsIndex_r4/Counter  cnt_type=Free Running  cnt_to=Inf  operation=Up  start_count=0  cnt_by_val=1  arith_type=Unsigned  n_bits=4  bin_pt=0  load_pin=off  rst=off  en=on  explicit_period=on  period=1  dbl_ovrd=off  use_behavioral_HDL=off  implementation=Fabric  block_type=counter
  Delay1 : xbsIndex_r4/Delay  rst=off  infoeditControl=Selection of Reset will increase slice count due to use of real FFs and instead of SRLs  en=on  latency=10  dbl_ovrd=off  reg_retiming=on  block_type=delay
  Expression1 : xbsIndex_r4/Expression  expression=a & b  align_bp=on  en=off  latency=0  precision=Full  arith_type=Unsigned  n_bits=16  bin_pt=0  dbl_ovrd=off  block_type=expr
  Relational1 : xbsIndex_r4/Relational  mode=a=b  en=off  latency=0  dbl_ovrd=off  block_type=relational
  Out1 : Outport
  wires:
  Valid/1 -> Counter1/1, Expression1/2
  Counter1/1 -> Relational1/1
  Const1/1 -> Relational1/2
  Relational1/1 -> Expression1/1
  Data/1 -> Delay1/1
  Expression1/1 -> Delay1/2
  Delay1/1 -> Out1/1

== system dedisp_sync/Parallel_Dedispersor_v6/Dedispersor_v2_2/detector_block_v2 ==
  Data : Inport
  Valid : Inport  Port=2
  Const1 : xbsIndex_r4/Constant  const=0  gui_display_data_type=Fixed-point  arith_type=Signed (2's comp)  n_bits=16  bin_pt=0  preci_type=Single  exp_width=8  frac_width=24  explicit_period=off  period=1  equ=P=C  opselect=C  inp2=PCIN>>17  opr=+  inp1=P  carry=CIN  dbl_ovrd=off  block_type=constant
  Counter1 : xbsIndex_r4/Counter  cnt_type=Free Running  cnt_to=Inf  operation=Up  start_count=0  cnt_by_val=1  arith_type=Unsigned  n_bits=4  bin_pt=0  load_pin=off  rst=off  en=on  explicit_period=on  period=1  dbl_ovrd=off  use_behavioral_HDL=off  implementation=Fabric  block_type=counter
  Delay1 : xbsIndex_r4/Delay  rst=off  infoeditControl=Selection of Reset will increase slice count due to use of real FFs and instead of SRLs  en=on  latency=1  dbl_ovrd=off  reg_retiming=on  block_type=delay
  Expression1 : xbsIndex_r4/Expression  expression=a & b  align_bp=on  en=off  latency=0  precision=Full  arith_type=Unsigned  n_bits=16  bin_pt=0  dbl_ovrd=off  block_type=expr
  Relational1 : xbsIndex_r4/Relational  mode=a=b  en=off  latency=0  dbl_ovrd=off  block_type=relational
  Out1 : Outport
  wires:
  Valid/1 -> Counter1/1, Expression1/2
  Counter1/1 -> Relational1/1
  Const1/1 -> Relational1/2
  Relational1/1 -> Expression1/1
  Data/1 -> Delay1/1
  Expression1/1 -> Delay1/2
  Delay1/1 -> Out1/1

== system dedisp_sync/Parallel_Dedispersor_v6/Dedispersor_v2_2/detector_block_v21 ==
  Data : Inport
  Valid : Inport  Port=2
  Const1 : xbsIndex_r4/Constant  const=1  gui_display_data_type=Fixed-point  arith_type=Signed (2's comp)  n_bits=16  bin_pt=0  preci_type=Single  exp_width=8  frac_width=24  explicit_period=off  period=1  equ=P=C  opselect=C  inp2=PCIN>>17  opr=+  inp1=P  carry=CIN  dbl_ovrd=off  block_type=constant
  Counter1 : xbsIndex_r4/Counter  cnt_type=Free Running  cnt_to=Inf  operation=Up  start_count=0  cnt_by_val=1  arith_type=Unsigned  n_bits=4  bin_pt=0  load_pin=off  rst=off  en=on  explicit_period=on  period=1  dbl_ovrd=off  use_behavioral_HDL=off  implementation=Fabric  block_type=counter
  Delay1 : xbsIndex_r4/Delay  rst=off  infoeditControl=Selection of Reset will increase slice count due to use of real FFs and instead of SRLs  en=on  latency=2  dbl_ovrd=off  reg_retiming=on  block_type=delay
  Expression1 : xbsIndex_r4/Expression  expression=a & b  align_bp=on  en=off  latency=0  precision=Full  arith_type=Unsigned  n_bits=16  bin_pt=0  dbl_ovrd=off  block_type=expr
  Relational1 : xbsIndex_r4/Relational  mode=a=b  en=off  latency=0  dbl_ovrd=off  block_type=relational
  Out1 : Outport
  wires:
  Valid/1 -> Counter1/1, Expression1/2
  Counter1/1 -> Relational1/1
  Const1/1 -> Relational1/2
  Relational1/1 -> Expression1/1
  Data/1 -> Delay1/1
  Expression1/1 -> Delay1/2
  Delay1/1 -> Out1/1

== system dedisp_sync/Parallel_Dedispersor_v6/Dedispersor_v2_2/detector_block_v210 ==
  Data : Inport
  Valid : Inport  Port=2
  Const1 : xbsIndex_r4/Constant  const=10  gui_display_data_type=Fixed-point  arith_type=Signed (2's comp)  n_bits=16  bin_pt=0  preci_type=Single  exp_width=8  frac_width=24  explicit_period=off  period=1  equ=P=C  opselect=C  inp2=PCIN>>17  opr=+  inp1=P  carry=CIN  dbl_ovrd=off  block_type=constant
  Counter1 : xbsIndex_r4/Counter  cnt_type=Free Running  cnt_to=Inf  operation=Up  start_count=0  cnt_by_val=1  arith_type=Unsigned  n_bits=4  bin_pt=0  load_pin=off  rst=off  en=on  explicit_period=on  period=1  dbl_ovrd=off  use_behavioral_HDL=off  implementation=Fabric  block_type=counter
  Delay1 : xbsIndex_r4/Delay  rst=off  infoeditControl=Selection of Reset will increase slice count due to use of real FFs and instead of SRLs  en=on  latency=11  dbl_ovrd=off  reg_retiming=on  block_type=delay
  Expression1 : xbsIndex_r4/Expression  expression=a & b  align_bp=on  en=off  latency=0  precision=Full  arith_type=Unsigned  n_bits=16  bin_pt=0  dbl_ovrd=off  block_type=expr
  Relational1 : xbsIndex_r4/Relational  mode=a=b  en=off  latency=0  dbl_ovrd=off  block_type=relational
  Out1 : Outport
  wires:
  Valid/1 -> Counter1/1, Expression1/2
  Counter1/1 -> Relational1/1
  Const1/1 -> Relational1/2
  Relational1/1 -> Expression1/1
  Data/1 -> Delay1/1
  Expression1/1 -> Delay1/2
  Delay1/1 -> Out1/1

== system dedisp_sync/Parallel_Dedispersor_v6/Dedispersor_v2_2/detector_block_v211 ==
  Data : Inport
  Valid : Inport  Port=2
  Const1 : xbsIndex_r4/Constant  const=11  gui_display_data_type=Fixed-point  arith_type=Signed (2's comp)  n_bits=16  bin_pt=0  preci_type=Single  exp_width=8  frac_width=24  explicit_period=off  period=1  equ=P=C  opselect=C  inp2=PCIN>>17  opr=+  inp1=P  carry=CIN  dbl_ovrd=off  block_type=constant
  Counter1 : xbsIndex_r4/Counter  cnt_type=Free Running  cnt_to=Inf  operation=Up  start_count=0  cnt_by_val=1  arith_type=Unsigned  n_bits=4  bin_pt=0  load_pin=off  rst=off  en=on  explicit_period=on  period=1  dbl_ovrd=off  use_behavioral_HDL=off  implementation=Fabric  block_type=counter
  Delay1 : xbsIndex_r4/Delay  rst=off  infoeditControl=Selection of Reset will increase slice count due to use of real FFs and instead of SRLs  en=on  latency=12  dbl_ovrd=off  reg_retiming=on  block_type=delay
  Expression1 : xbsIndex_r4/Expression  expression=a & b  align_bp=on  en=off  latency=0  precision=Full  arith_type=Unsigned  n_bits=16  bin_pt=0  dbl_ovrd=off  block_type=expr
  Relational1 : xbsIndex_r4/Relational  mode=a=b  en=off  latency=0  dbl_ovrd=off  block_type=relational
  Out1 : Outport
  wires:
  Valid/1 -> Counter1/1, Expression1/2
  Counter1/1 -> Relational1/1
  Const1/1 -> Relational1/2
  Relational1/1 -> Expression1/1
  Data/1 -> Delay1/1
  Expression1/1 -> Delay1/2
  Delay1/1 -> Out1/1

== system dedisp_sync/Parallel_Dedispersor_v6/Dedispersor_v2_2/detector_block_v212 ==
  Data : Inport
  Valid : Inport  Port=2
  Const1 : xbsIndex_r4/Constant  const=12  gui_display_data_type=Fixed-point  arith_type=Signed (2's comp)  n_bits=16  bin_pt=0  preci_type=Single  exp_width=8  frac_width=24  explicit_period=off  period=1  equ=P=C  opselect=C  inp2=PCIN>>17  opr=+  inp1=P  carry=CIN  dbl_ovrd=off  block_type=constant
  Counter1 : xbsIndex_r4/Counter  cnt_type=Free Running  cnt_to=Inf  operation=Up  start_count=0  cnt_by_val=1  arith_type=Unsigned  n_bits=4  bin_pt=0  load_pin=off  rst=off  en=on  explicit_period=on  period=1  dbl_ovrd=off  use_behavioral_HDL=off  implementation=Fabric  block_type=counter
  Delay1 : xbsIndex_r4/Delay  rst=off  infoeditControl=Selection of Reset will increase slice count due to use of real FFs and instead of SRLs  en=on  latency=13  dbl_ovrd=off  reg_retiming=on  block_type=delay
  Expression1 : xbsIndex_r4/Expression  expression=a & b  align_bp=on  en=off  latency=0  precision=Full  arith_type=Unsigned  n_bits=16  bin_pt=0  dbl_ovrd=off  block_type=expr
  Relational1 : xbsIndex_r4/Relational  mode=a=b  en=off  latency=0  dbl_ovrd=off  block_type=relational
  Out1 : Outport
  wires:
  Valid/1 -> Counter1/1, Expression1/2
  Counter1/1 -> Relational1/1
  Const1/1 -> Relational1/2
  Relational1/1 -> Expression1/1
  Data/1 -> Delay1/1
  Expression1/1 -> Delay1/2
  Delay1/1 -> Out1/1

== system dedisp_sync/Parallel_Dedispersor_v6/Dedispersor_v2_2/detector_block_v213 ==
  Data : Inport
  Valid : Inport  Port=2
  Const1 : xbsIndex_r4/Constant  const=13  gui_display_data_type=Fixed-point  arith_type=Signed (2's comp)  n_bits=16  bin_pt=0  preci_type=Single  exp_width=8  frac_width=24  explicit_period=off  period=1  equ=P=C  opselect=C  inp2=PCIN>>17  opr=+  inp1=P  carry=CIN  dbl_ovrd=off  block_type=constant
  Counter1 : xbsIndex_r4/Counter  cnt_type=Free Running  cnt_to=Inf  operation=Up  start_count=0  cnt_by_val=1  arith_type=Unsigned  n_bits=4  bin_pt=0  load_pin=off  rst=off  en=on  explicit_period=on  period=1  dbl_ovrd=off  use_behavioral_HDL=off  implementation=Fabric  block_type=counter
  Delay1 : xbsIndex_r4/Delay  rst=off  infoeditControl=Selection of Reset will increase slice count due to use of real FFs and instead of SRLs  en=on  latency=14  dbl_ovrd=off  reg_retiming=on  block_type=delay
  Expression1 : xbsIndex_r4/Expression  expression=a & b  align_bp=on  en=off  latency=0  precision=Full  arith_type=Unsigned  n_bits=16  bin_pt=0  dbl_ovrd=off  block_type=expr
  Relational1 : xbsIndex_r4/Relational  mode=a=b  en=off  latency=0  dbl_ovrd=off  block_type=relational
  Out1 : Outport
  wires:
  Valid/1 -> Counter1/1, Expression1/2
  Counter1/1 -> Relational1/1
  Const1/1 -> Relational1/2
  Relational1/1 -> Expression1/1
  Data/1 -> Delay1/1
  Expression1/1 -> Delay1/2
  Delay1/1 -> Out1/1
